simulink model "Reponses_Simulink"  (R2019a)
settings: Solver=VariableStepAuto  StartTime=0.0  StopTime=2  RelTol=1e-3
settings Model: Creator=Andre  LastModifiedBy=Andre

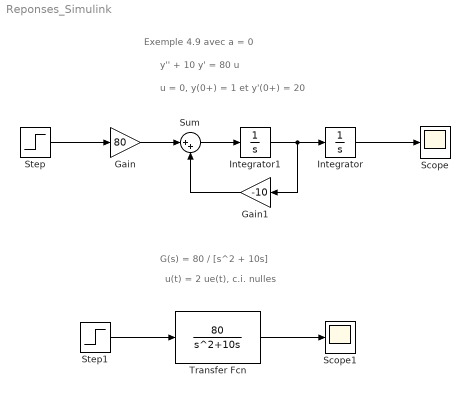
== system Reponses_Simulink ==
  note: y'' + 10 y' = 80 u
  note: Exemple 4.9 avec a = 0
  note: u = 0, y(0+) = 1 et y'(0+) = 20
  note: G(s) = 80 / [s^2 + 10s]
  note: u(t) = 2 ue(t), c.i. nulles
  Gain : Gain  Gain=80
  Gain1 : Gain  Gain=-10
  Integrator : Integrator  InitialCondition=1
  Integrator1 : Integrator  InitialCondition=20
  Scope : Scope
  Scope1 : Scope
  Step : Step  Time=0  After=0  SampleTime=0
  Step1 : Step  Time=0  After=2  SampleTime=0
  Sum : Sum  Inputs=|++
  Transfer Fcn : TransferFcn  Numerator=[80]  Denominator=[1 10 0]
  wires:
  Integrator1/1 -> Gain1/1, Integrator/1
  Sum/1 -> Integrator1/1
  Gain/1 -> Sum/1
  Gain1/1 -> Sum/2
  Step/1 -> Gain/1
  Integrator/1 -> Scope/1
  Step1/1 -> Transfer Fcn/1
  Transfer Fcn/1 -> Scope1/1
